simulink model "w11"  (R2024a)
settings: Solver=VariableStepAuto  StartTime=0.0  StopTime=1  MaxStep=1e-4  RelTol=1e-3
values from neighbouring files (symbols this model uses):
  B = 0.0001    [main.m]
  J = 0.045    [main.m]
  Lamf = 0.12    [main.m]
  Lds = 30.0e-3    (= 0.03)    [main.m]
  Lqs = 30.0e-3    (= 0.03)    [main.m]
  P = 24    [main.m]
  Rs = 2    [main.m]
  TL = 20    [main.m]
settings Model: Creator=moon  LastModifiedBy=moon
settings RTWCC: GPUComputeCapability=3.5

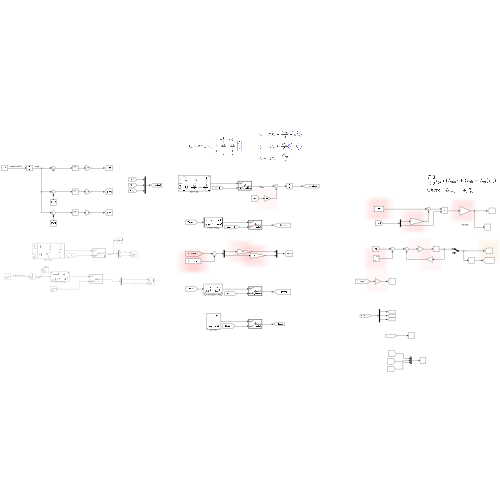
[thumbnail: Simulink's stored preview of the top-level diagram]
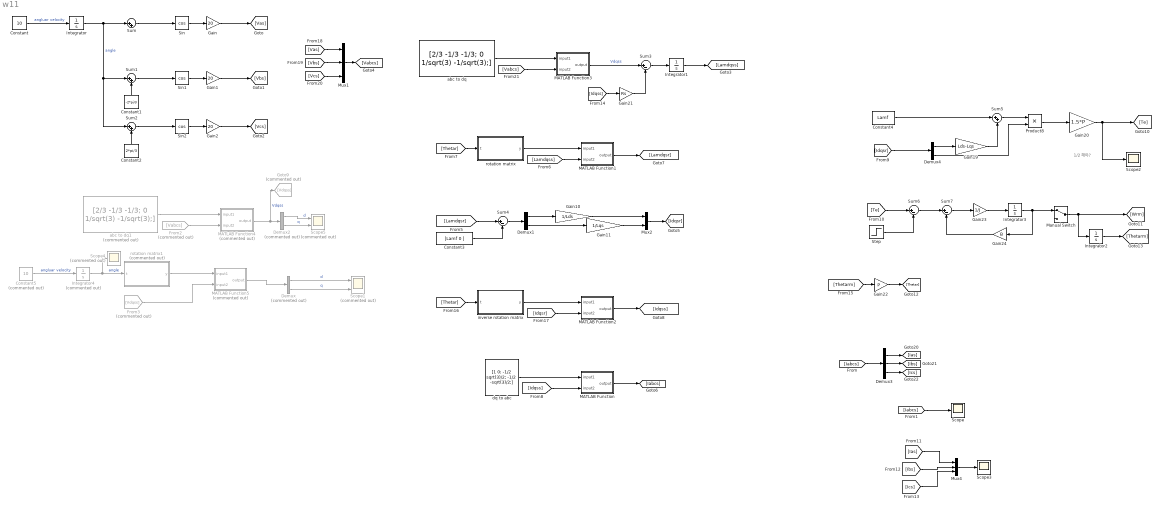
== system w11 ==
  note: 1/2 해야?
  Constant : Constant  Value=10
  Constant1 : Constant  Value=-2*pi/3
  Constant2 : Constant  Value=2*pi/3
  Constant3 : Constant  Value=[Lamf 0 ]
  Constant4 : Constant  Value=Lamf
  Constant5 : Constant  Commented=on  Value=10
  Demux : Demux  Commented=on  Outputs=2
  Demux1 : Demux  Outputs=2
  Demux2 : Demux  Commented=on  Outputs=2
  Demux3 : Demux  Outputs=3
  Demux4 : Demux  Outputs=2
  From2 : From  Commented=on  GotoTag=Vabcs
  From3 : From  Commented=on  GotoTag=Vdqss
  Gain : Gain  Gain=20
  Gain1 : Gain  Gain=20
  Gain10 : Gain  Gain=1/Lds
  Gain11 : Gain  Gain=1/Lqs
  Gain19 : Gain  Gain=Lds-Lqs
  Gain2 : Gain  Gain=20
  Gain20 : Gain  Gain=1.5*P
  Gain21 : Gain  Gain=Rs
  Gain22 : Gain  Gain=P
  Gain23 : Gain  Gain=1/J
  Gain24 : Gain  Gain=B
  Goto9 : Goto  Commented=on  GotoTag=Vdqss
  Integrator{,1..3} (4 alike) : Integrator
  Integrator4 : Integrator  Commented=on
  MATLAB Function : MATLAB Function  TreatAsAtomicUnit=on
  MATLAB Function1 : MATLAB Function  TreatAsAtomicUnit=on
  MATLAB Function2 : MATLAB Function  TreatAsAtomicUnit=on
  MATLAB Function3 : MATLAB Function  TreatAsAtomicUnit=on
  MATLAB Function4 : MATLAB Function  Commented=on  TreatAsAtomicUnit=on
  MATLAB Function5 : MATLAB Function  Commented=on  TreatAsAtomicUnit=on
  Manual Switch : ManualSwitch
  Mux1 : Mux  Inputs=3
  Mux2 : Mux  Inputs=2
  Mux4 : Mux  Inputs=3
  Product8 : Product
  Scope : Scope
  Scope1 : Scope  Commented=on  NumInputPorts=2
  Scope2 : Scope
  Scope3 : Scope
  Scope4 : Scope  Commented=on
  Scope5 : Scope  Commented=on  NumInputPorts=2
  Sin : Trigonometry  Operator=cos
  Sin1 : Trigonometry  Operator=cos
  Sin2 : Trigonometry  Operator=cos
  Step : Step  Time=0.5  After=TL  SampleTime=0
  Sum{,1..2,5} (4 alike) : Sum  Inputs=|++
  Sum{3..4,6..7} (4 alike) : Sum  Inputs=|+-
  abc to dq : Constant  Value=[2/3 -1/3 -1/3; 0 1/sqrt(3) -1/sqrt(3);]
      mask Display: image(imread('img/abc2dq.png'))
  abc to dq1 : Constant  Commented=on  Value=[2/3 -1/3 -1/3; 0 1/sqrt(3) -1/sqrt(3);]
      mask Display: image(imread('img/abc2dq.png'))
  dq to abc : Constant  Value=[1 0; -1/2 sqrt(3)/2; -1/2 -sqrt(3)/2;]
      mask Display: image(imread('img/dq2abc.png'))
  inverse rotation matrix : Subsystem
      mask Display: image(imread('img/rotateMatrix.png'))
  rotation matrix : Subsystem
      mask Display: image(imread('img/rotateInverseMatrix.png'))
  rotation matrix1 : Subsystem  Commented=on
      mask Display: image(imread('img/rotateInverseMatrix.png'))
  wires:
  Gain/1 -> [Vas]
  Sin/1 -> Gain/1
  Sum/1 -> Sin/1
  Constant/1 -> Integrator/1  "angluar velocity"
  Sin1/1 -> Gain1/1
  Gain1/1 -> [Vbs]
  Sum1/1 -> Sin1/1
  Gain2/1 -> [Vcs]
  Sum2/1 -> Sin2/1
  Sin2/1 -> Gain2/1
  Integrator/1 -> Sum2/1, Sum1/1, Sum/1  "angle"
  Constant1/1 -> Sum1/2
  Constant2/1 -> Sum2/2
  Sum3/1 -> Integrator1/1
  Integrator1/1 -> [Lamdqss]
  MATLAB Function3/1(output) -> Sum3/1  "Vdqss"
  [Lamdqsr] -> Sum4/1
  Constant3/1 -> Sum4/2
  Sum4/1 -> Demux1/1
  Demux1/1 -> Gain10/1
  Demux1/2 -> Gain11/1
  Gain10/1 -> Mux2/1
  Gain11/1 -> Mux2/2
  Mux2/1 -> [Idqsr]
  [Idqsr] -> Demux4/1
  Demux4/1 -> Gain19/1
  Constant4/1 -> Sum5/1
  Gain19/1 -> Sum5/2
  Sum5/1 -> Product8/1
  Demux4/2 -> Product8/2
  Product8/1 -> Gain20/1
  Gain20/1 -> Scope2/1, [Te]
  [Te] -> Sum6/1
  Sum6/1 -> Sum7/1
  Integrator3/1 -> Manual Switch/1, Gain24/1
  Step/1 -> Sum6/2
  [Ias] -> Mux4/1
  [Ibs] -> Mux4/2
  [Ics] -> Mux4/3
  Mux4/1 -> Scope3/1
  [Idqss] -> Gain21/1
  Gain21/1 -> Sum3/2
  Gain22/1 -> [Thetar]
  [Thetarm] -> Gain22/1
  Integrator2/1 -> [Thetarm]
  Sum7/1 -> Gain23/1
  Gain23/1 -> Integrator3/1
  Gain24/1 -> Sum7/2
  dq to abc/1 -> MATLAB Function/1(input1)
  [Idqss] -> MATLAB Function/2(input2)
  MATLAB Function/1(output) -> [Iabcs]
  Demux3/1 -> [Ias]
  Demux3/2 -> [Ibs]
  Demux3/3 -> [Ics]
  [Lamdqss] -> MATLAB Function1/2(input2)
  MATLAB Function1/1(output) -> [Lamdqsr]
  [Thetar] -> rotation matrix/1(t)
  rotation matrix/1(y) -> MATLAB Function1/1(input1)
  MATLAB Function2/1(output) -> [Idqss]
  [Thetar] -> inverse rotation matrix/1(t)
  inverse rotation matrix/1(y) -> MATLAB Function2/1(input1)
  [Idqsr] -> MATLAB Function2/2(input2)
  abc to dq/1 -> MATLAB Function3/1(input1)
  [Vabcs] -> MATLAB Function3/2(input2)
  [Vas] -> Mux1/1
  [Vbs] -> Mux1/2
  [Vcs] -> Mux1/3
  Mux1/1 -> [Vabcs]
  Manual Switch/1 -> Integrator2/1, [Wrm]
  [Iabcs] -> Demux3/1
  [Iabcs] -> Scope/1
  abc to dq1/1 -> MATLAB Function4/1(input1)
  From2/1 -> MATLAB Function4/2(input2)
  MATLAB Function4/1(output) -> Goto9/1, Demux2/1  "Vdqss"
  Constant5/1 -> Integrator4/1  "angluar velocity"
  Integrator4/1 -> Scope4/1, rotation matrix1/1(t)  "angle"
  rotation matrix1/1(y) -> MATLAB Function5/1(input1)
  From3/1 -> MATLAB Function5/2(input2)
  MATLAB Function5/1(output) -> Demux/1
  Demux/1 -> Scope1/1  "d"
  Demux/2 -> Scope1/2  "q"
  Demux2/1 -> Scope5/1  "d"
  Demux2/2 -> Scope5/2  "q"

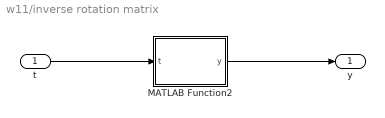
== system w11/inverse rotation matrix ==
  t : Inport
  MATLAB Function2 : MATLAB Function  TreatAsAtomicUnit=on
  y : Outport
  wires:
  MATLAB Function2/1(y) -> y/1
  t/1 -> MATLAB Function2/1(t)

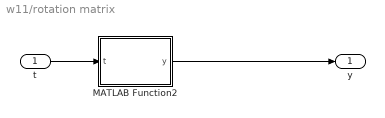
== system w11/rotation matrix ==
  t : Inport
  MATLAB Function2 : MATLAB Function  TreatAsAtomicUnit=on
  y : Outport
  wires:
  MATLAB Function2/1(y) -> y/1
  t/1 -> MATLAB Function2/1(t)

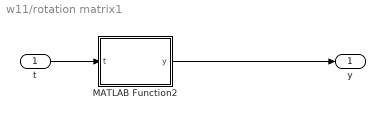
== system w11/rotation matrix1 ==
  t : Inport
  MATLAB Function2 : MATLAB Function  TreatAsAtomicUnit=on
  y : Outport
  wires:
  MATLAB Function2/1(y) -> y/1
  t/1 -> MATLAB Function2/1(t)

== matlab function w11/MATLAB Function ==
  data: input1 input; output output; input2 input
function output = matrix_multiply(input1, input2)
    % 행렬 곱셈 (input1의 열 수 = input2의 행 수)
    output = input1 * input2;
end

== matlab function w11/rotation matrix/MATLAB Function2 ==
  data: t input; y output
function y = matrix_output(t)
y = [cos(t) sin(t); -sin(t) cos(t)];

== matlab function w11/MATLAB Function2 ==
  data: input1 input; output output; input2 input
function output = matrix_multiply(input1, input2)
    % 행렬 곱셈 (input1의 열 수 = input2의 행 수)
    output = input1 * input2;
end

== matlab function w11/inverse rotation matrix/MATLAB Function2 ==
  data: t input; y output
function y = matrix_output(t)
y = [cos(t) -sin(t); sin(t) cos(t)];

== matlab function w11/MATLAB Function3 ==
  data: input1 input; output output; input2 input
function output = matrix_multiply(input1, input2)
    % 행렬 곱셈 (input1의 열 수 = input2의 행 수)
    output = input1 * input2;
end

== matlab function w11/MATLAB Function4 ==
  data: input1 input; output output; input2 input
function output = matrix_multiply(input1, input2)
    % 행렬 곱셈 (input1의 열 수 = input2의 행 수)
    output = input1 * input2;
end

== matlab function w11/rotation matrix1/MATLAB Function2 ==
  data: t input; y output
function y = matrix_output(t)
y = [cos(t) sin(t); -sin(t) cos(t)];

== matlab function w11/MATLAB Function5 ==
  data: input1 input; output output; input2 input
function output = matrix_multiply(input1, input2)
    % 행렬 곱셈 (input1의 열 수 = input2의 행 수)
    output = input1 * input2;
end

== matlab function w11/MATLAB Function1 ==
  data: input1 input; output output; input2 input
function output = matrix_multiply(input1, input2)
    % 행렬 곱셈 (input1의 열 수 = input2의 행 수)
    output = input1 * input2;
end
